simulink model "px4demo_attitude_system20190504_pitch"  (R2016b)
settings: Solver=FixedStepDiscrete  StartTime=0.0  StopTime=inf  RelTol=1e-3
PostLoadFcn:
  | kFactor = 1.2;
  | 
  | KpRollAttitude = 0.630138625117681 / kFactor;
  | KiRollAttitude = 0.0552303199591522 / kFactor;
  | 
  | KpPitchAttitude = 0.630138625117681 / kFactor;
  | KiPitchAttitude = 0.0552303199591522 / kFactor;
  | 
  | KpRollRate = 1.31533836563383 / kFactor;
  | KiRollRate = 0.460338699849681 / kFactor;
  | 
  | KpPitchRate = 1.31533836563383 / kFactor;
  | KiPitchRate = 0.460338699849681 / kFactor;
  | 
  | KpYawRate = 1.31533836563383 / kFactor;
  | KiYawRate = 0.460338699849681 / kFactor;
undefined symbols (not defined in the file or in its folder): PX4_TUNE_ENUM, RGBLED_COLOR_ENUM, RGBLED_MODE_ENUM
libraries: pixhawk_slib_sensors_actuators x7, pixhawk_slib_ADC_serial x1, pixhawk_slib_misc_utils x1, pixhawk_slib_uORB_RW x1
settings Model: Creator=Steve  LastModifiedBy=DELL
settings SolverCC: AutoInsertRateTranBlk=on
settings DataIOCC: LimitDataPoints=on  SaveFormat=Array
settings OptimizationCC: DefaultParameterBehavior=Inlined  LifeSpan=1  MaxStackSize=64
settings DebuggingCC: SolverPrmCheckMsg=warning  AllowSymbolicDim=off  SFUnexpectedBacktrackingDiag=warning  SFNoUnconditionalDefaultTransitionDiag=warning  SFExecutionAtInitializationDiag=none
settings HardwareCC: ProdBitPerPointer=32  ProdBitPerSizeT=32  ProdBitPerPtrDiffT=32  ProdLargestAtomicInteger=Long  ProdLargestAtomicFloat=Double  ProdWordSize=32  ProdHWDeviceType=ARM Compatible->ARM Cortex
settings ModelReferenceCC: PropagateSignalLabelsOutOfModel=off
settings RTWCC: SystemTargetFile=ert.tlc  HardwareBoard=Pixhawk PX4  TemplateMakefile=ert_default_tmf  Description=Embedded Coder  GenerateReport=on  Toolchain=Pixhawk Toolchain  IncludeHyperlinkInReport=on  LaunchReport=on  GenerateTraceReport=on  GenerateTraceReportSl=on  GenerateTraceReportSf=on  GenerateTraceReportEml=on  GenerateCodeMetricsReport=on
settings CodeAppCC: IgnoreCustomStorageClasses=off
settings ERTTargetCC: CodeReplacementLibrary=GCC ARM Cortex-A9  ExtModeTransport=1  ExtModeMexFile=ext_serial_win32_comm  ExtModeMexArgs=/dev/serial  ERTCustomFileTemplate=PX4_codertarget_file_process.tlc  ConvertIfToSwitch=off  SuppressUnreachableDefaultCases=off
settings ConfigComp: CovMetricSettings=dw  CovHtmlReporting=on  CovSaveCumulativeToWorkspaceVar=on  CovSaveSingleToWorkspaceVar=on  CovExternalEMLEnable=off  CovSFcnEnable=off

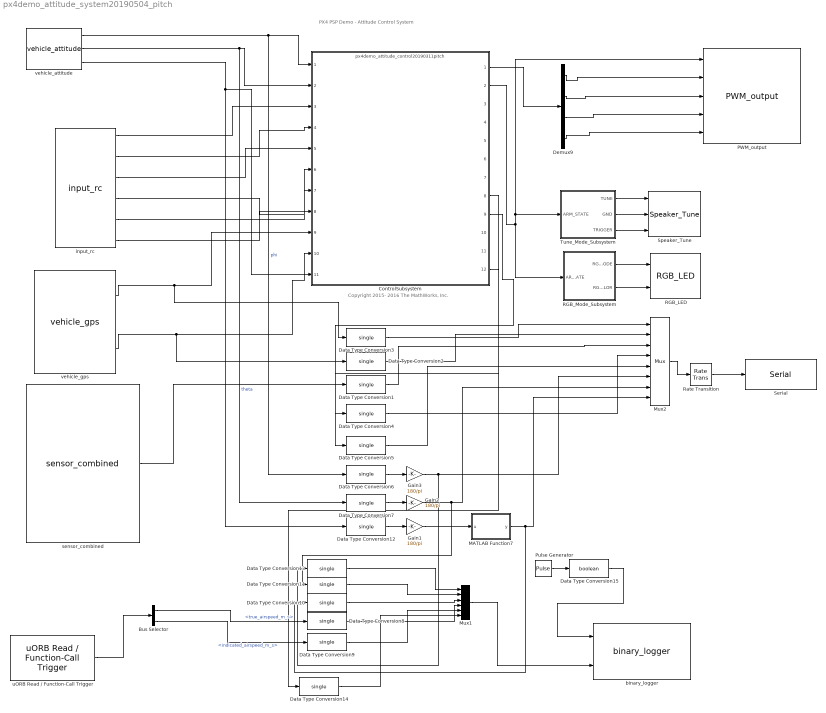
== system px4demo_attitude_system20190504_pitch ==
  note: PX4 PSP Demo - Attitude Control System
  note: Copyright 2015- 2016 The MathWorks, Inc.
  Bus Selector : BusSelector  OutputSignals=true_airspeed_m_s,indicated_airspeed_m_s
  ControlSubsystem : ModelReference  ModelNameDialog=px4demo_attitude_control20190311pitch.slx  SimulationMode=Normal  ModelReferenceVersion=1.389
  Data Type Conversion{1..14} (14 alike) : DataTypeConversion  OutDataTypeStr=single
  Data Type Conversion15 : DataTypeConversion  OutDataTypeStr=boolean
  Demux9 : Demux
  Gain1 : Gain  Gain=180/pi
  Gain2 : Gain  Gain=180/pi
  Gain3 : Gain  Gain=180/pi
  MATLAB Function7 : MATLAB Function  TreatAsAtomicUnit=on
  Mux1 : Mux  Inputs=6
  Mux2 : Mux  Inputs=8
  PWM_output : pixhawk_slib_sensors_actuators/PWM_output  pwm_rate=50Hz  show_pwm1=on  show_pwm2=on  show_pwm3=on  show_pwm4=on  show_pwm5=off  show_pwm6=off  show_pwm7=off  show_pwm8=off
  Pulse Generator : DiscretePulseGenerator  Period=10  PulseWidth=5  SampleTime=10
  RGB_LED : pixhawk_slib_sensors_actuators/RGB_LED
  RGB_Mode_Subsystem : Subsystem
  Rate Transition : RateTransition  OutPortSampleTime=0.3
  Serial : pixhawk_slib_ADC_serial/Serial  DeviceName=/dev/ttyS1  ReadOrWrite=Writing  BaudRateStr=57600  block=on  WriteStatus=on  Terminator=off  Header=off  NumBytesRead=4  TerminatorChar=\n  HeaderData=57600  SimulateUsing=Code generation
  Speaker_Tune : pixhawk_slib_sensors_actuators/Speaker_Tune
  Tune_Mode_Subsystem : Subsystem
  binary_logger : pixhawk_slib_misc_utils/binary_logger  logfile=/fs/microsd/log  cacheflag=off  numRecs=1000
  input_rc : pixhawk_slib_sensors_actuators/input_rc  sampletime=1/250  channel1=on  channel2=on  channel3=on  channel4=on  channel5=on  channel6=on  channel7=off  channel8=off  ch_count=off  rssi=off  rc_failsafe=off  rc_lost=off  rc_inputsource=off
  sensor_combined : pixhawk_slib_sensors_actuators/sensor_combined  sampletime=1/250  show_mag=off  show_acc=off  show_gyro=off  show_baro=on  show_ts=off
  uORB Read / Function-Call Trigger : pixhawk_slib_uORB_RW/uORB Read // Function-Call Trigger  uORB_Topic_str='airspeed'  BusObjVar=Bus: airspeed_SL  uORB_Interval=1  AsyncOutput=off  Fcn_call_select=Generate Function Call Signal  TaskName='Task1'  Poll_timeout=100  Ts=-1
  vehicle_attitude : pixhawk_slib_sensors_actuators/vehicle_attitude  sampletime=1/250  show_r=on  show_p=on  show_y=on  show_q=off
  vehicle_gps : pixhawk_slib_sensors_actuators/vehicle_gps  sampletime=1/250  show_ts_pos=off  show_alt=off  show_ts_gps=off  show_vel=off  show_fixtype=off  show_numsat=off
  wires:
  Demux9/4 -> PWM_output/5
  Demux9/2 -> PWM_output/3
  Demux9/3 -> PWM_output/4
  Demux9/1 -> PWM_output/2
  RGB_Mode_Subsystem/1(RGB_MODE) -> RGB_LED/1
  RGB_Mode_Subsystem/2(RGB_COLOR) -> RGB_LED/2
  Tune_Mode_Subsystem/1(TUNE) -> Speaker_Tune/1
  Tune_Mode_Subsystem/2(GND) -> Speaker_Tune/2
  Tune_Mode_Subsystem/3(TRIGGER) -> Speaker_Tune/3
  ControlSubsystem/2 -> Tune_Mode_Subsystem/1(ARM_STATE), PWM_output/1, RGB_Mode_Subsystem/1(ARM_STATE)
  vehicle_attitude/1 -> Data Type Conversion6/1, ControlSubsystem/1  "phi"
  vehicle_attitude/2 -> Data Type Conversion7/1, ControlSubsystem/2  "theta"
  input_rc/1 -> ControlSubsystem/3
  input_rc/2 -> ControlSubsystem/4
  input_rc/3 -> ControlSubsystem/5
  input_rc/4 -> ControlSubsystem/6
  input_rc/5 -> ControlSubsystem/7
  ControlSubsystem/1 -> Demux9/1
  input_rc/6 -> ControlSubsystem/8
  Rate Transition/1 -> Serial/1
  Mux2/1 -> Rate Transition/1
  vehicle_gps/1 -> Data Type Conversion3/1, ControlSubsystem/9
  vehicle_gps/2 -> Data Type Conversion2/1, ControlSubsystem/10
  Data Type Conversion12/1 -> Gain1/1
  vehicle_attitude/3 -> ControlSubsystem/11, Data Type Conversion12/1
  Gain1/1 -> MATLAB Function7/1(u)
  sensor_combined/1 -> Data Type Conversion1/1
  Data Type Conversion3/1 -> Mux2/1
  Data Type Conversion2/1 -> Mux2/2
  Data Type Conversion1/1 -> Mux2/3
  ControlSubsystem/8 -> Data Type Conversion4/1
  Data Type Conversion4/1 -> Mux2/4
  ControlSubsystem/9 -> Data Type Conversion5/1
  Data Type Conversion5/1 -> Mux2/5
  Data Type Conversion6/1 -> Gain3/1
  Data Type Conversion7/1 -> Gain2/1
  Gain3/1 -> Data Type Conversion13/1, Mux2/6
  Gain2/1 -> Data Type Conversion11/1, Mux2/7
  MATLAB Function7/1(y) -> Data Type Conversion10/1, Mux2/8
  Mux1/1 -> binary_logger/2
  Data Type Conversion8/1 -> Mux1/4
  uORB Read / Function-Call Trigger/1 -> Bus Selector/1
  Data Type Conversion9/1 -> Mux1/5
  Bus Selector/2 -> Data Type Conversion9/1  "<indicated_airspeed_m_s>"
  Bus Selector/1 -> Data Type Conversion8/1  "<true_airspeed_m_s>"
  Data Type Conversion10/1 -> Mux1/3
  Data Type Conversion11/1 -> Mux1/2
  Data Type Conversion13/1 -> Mux1/1
  Data Type Conversion14/1 -> Mux1/6
  ControlSubsystem/12 -> Data Type Conversion14/1
  Data Type Conversion15/1 -> binary_logger/1
  Pulse Generator/1 -> Data Type Conversion15/1

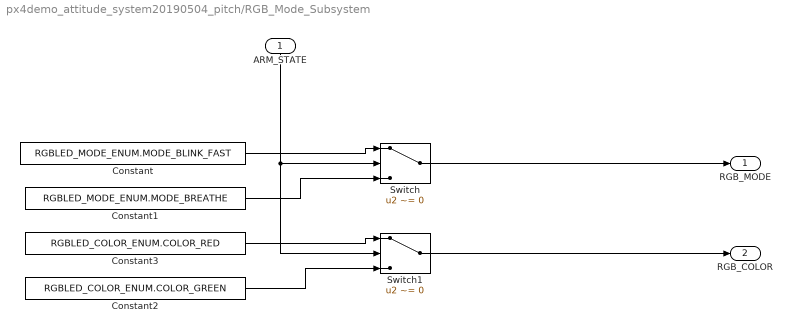
== system px4demo_attitude_system20190504_pitch/RGB_Mode_Subsystem ==
  ARM_STATE : Inport
  Constant : Constant  Value=RGBLED_MODE_ENUM.MODE_BLINK_FAST  OutDataTypeStr=Enum: RGBLED_MODE_ENUM
  Constant1 : Constant  Value=RGBLED_MODE_ENUM.MODE_BREATHE  OutDataTypeStr=Enum: RGBLED_MODE_ENUM
  Constant2 : Constant  Value=RGBLED_COLOR_ENUM.COLOR_GREEN  OutDataTypeStr=Enum: RGBLED_COLOR_ENUM
  Constant3 : Constant  Value=RGBLED_COLOR_ENUM.COLOR_RED  OutDataTypeStr=Enum: RGBLED_COLOR_ENUM
  Switch : Switch  Criteria=u2 ~= 0  Threshold=1500  SampleTime=1/2
  Switch1 : Switch  Criteria=u2 ~= 0  Threshold=1500  SampleTime=1/2
  RGB_MODE : Outport
  RGB_COLOR : Outport  Port=2
  wires:
  ARM_STATE/1 -> Switch1/2, Switch/2
  Constant/1 -> Switch/1
  Constant1/1 -> Switch/3
  Switch/1 -> RGB_MODE/1
  Constant3/1 -> Switch1/1
  Constant2/1 -> Switch1/3
  Switch1/1 -> RGB_COLOR/1

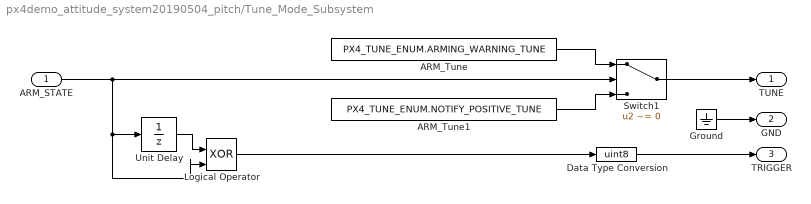
== system px4demo_attitude_system20190504_pitch/Tune_Mode_Subsystem ==
  ARM_STATE : Inport
  ARM_Tune : Constant  Value=PX4_TUNE_ENUM.ARMING_WARNING_TUNE  OutDataTypeStr=Enum: PX4_TUNE_ENUM
  ARM_Tune1 : Constant  Value=PX4_TUNE_ENUM.NOTIFY_POSITIVE_TUNE  OutDataTypeStr=Enum: PX4_TUNE_ENUM
  Data Type Conversion : DataTypeConversion  OutDataTypeStr=uint8
  Ground : Ground
  Logical Operator : Logic  Operator=XOR  IconShape=distinctive  AllPortsSameDT=off  OutDataTypeStr=boolean
  Switch1 : Switch  Criteria=u2 ~= 0  Threshold=1500
  Unit Delay : UnitDelay  SampleTime=-1
  TUNE : Outport
  GND : Outport  Port=2
  TRIGGER : Outport  Port=3
  wires:
  Ground/1 -> GND/1
  Data Type Conversion/1 -> TRIGGER/1
  Switch1/1 -> TUNE/1
  ARM_Tune/1 -> Switch1/1
  ARM_Tune1/1 -> Switch1/3
  ARM_STATE/1 -> Logical Operator/2, Unit Delay/1, Switch1/2
  Unit Delay/1 -> Logical Operator/1
  Logical Operator/1 -> Data Type Conversion/1

== matlab function px4demo_attitude_system20190504_pitch/MATLAB Function7 ==
  data: u input; y output
function y = fcn(u)
if(u<=0)
    y=360+u;
else
    y=u
end
